simulink model "Mrinal_230929228_Simulink"  (R2025a)
settings: Solver=VariableStepAuto  StartTime=0.0  StopTime=5  RelTol=1e-3
libraries: spsSeriesRLCBranchLib x12, spsMeanLib x11, spsCurrentMeasurementLib x7, spsDCVoltageSourceLib x5, spsVoltageMeasurementLib x5, spsIdealSwitchLib x4, spspowerguiLib x4, spsDiodeLib x3, simulink x1, sps_lib x1
settings Model: Creator=MRINAL  LastModifiedBy=MRINAL

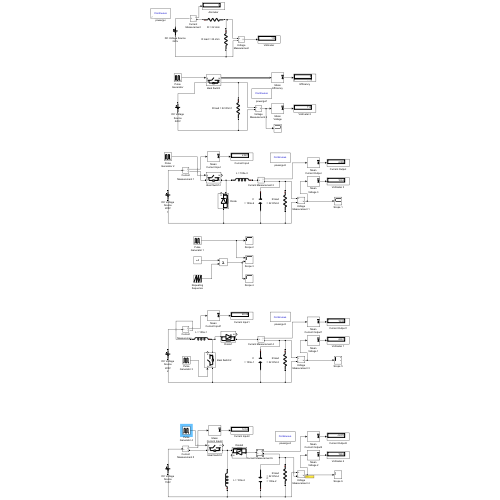
[thumbnail: Simulink's stored preview of the top-level diagram]
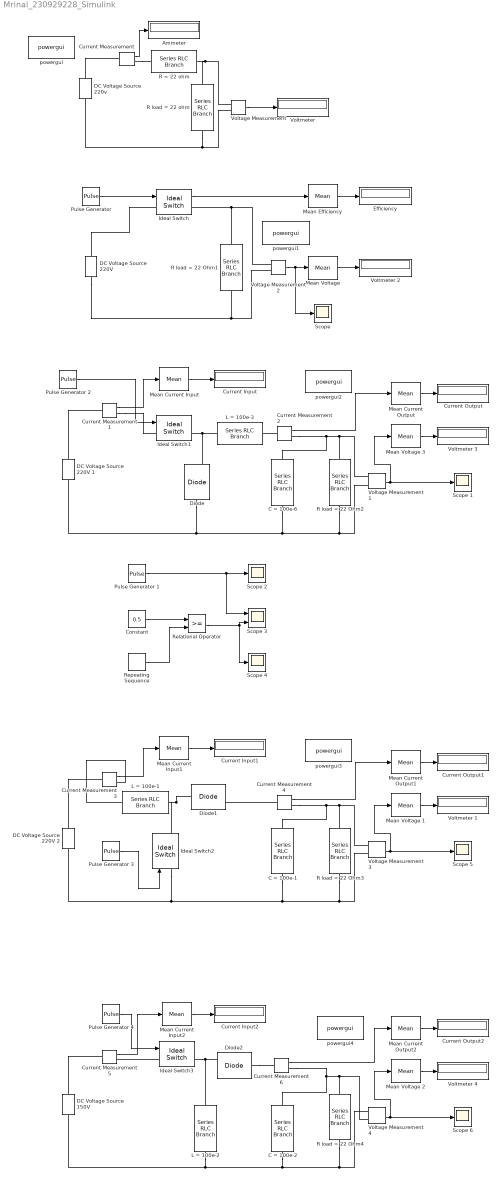
== system Mrinal_230929228_Simulink ==
  Ammeter : Display
  C = 100e-1 : spsSeriesRLCBranchLib/Series RLC Branch  LConnTagsString=__new0  RConnTagsString=__new0  BranchType=C  Resistance=22  Inductance=1e-3  SetiL0=off  InitialCurrent=0  Capacitance=100e-6  Setx0=off  InitialVoltage=0  Measurements=None
  C = 100e-2 : spsSeriesRLCBranchLib/Series RLC Branch  LConnTagsString=__new0  RConnTagsString=__new0  BranchType=C  Resistance=22  Inductance=1e-3  SetiL0=off  InitialCurrent=0  Capacitance=100e-6  Setx0=off  InitialVoltage=0  Measurements=None
  C = 100e-6 : spsSeriesRLCBranchLib/Series RLC Branch  LConnTagsString=__new0  RConnTagsString=__new0  BranchType=C  Resistance=22  Inductance=1e-3  SetiL0=off  InitialCurrent=0  Capacitance=100e-6  Setx0=off  InitialVoltage=0  Measurements=None
  Constant : Constant  Value=0.5
  Current Measurement : spsCurrentMeasurementLib/Current Measurement  PhasorSimulation=off  OutputType=Complex  PSBequivalent=0
  Current Measurement {1..6} (6 alike) : spsCurrentMeasurementLib/Current Measurement  PhasorSimulation=off  OutputType=Complex  PSBequivalent=0
  Current Input : Display
  Current Input1 : Display
  Current Input2 : Display
  Current Output : Display
  Current Output1 : Display
  Current Output2 : Display
  DC Voltage Source 150V : spsDCVoltageSourceLib/DC Voltage Source  Amplitude=150  Measurements=None
  DC Voltage Source 220V : spsDCVoltageSourceLib/DC Voltage Source  Amplitude=220  Measurements=None
  DC Voltage Source 220V 1 : spsDCVoltageSourceLib/DC Voltage Source  Amplitude=220  Measurements=None
  DC Voltage Source 220V 2 : spsDCVoltageSourceLib/DC Voltage Source  Amplitude=220  Measurements=None
  DC Voltage Source 220v : spsDCVoltageSourceLib/DC Voltage Source  Amplitude=220  Measurements=None
  Diode : spsDiodeLib/Diode  Ron=0.001  Lon=0  Vf=0.8  IC=0  UseSnubber=0  Rs=500  Cs=250e-9  Measurements=on
  Diode1 : spsDiodeLib/Diode  Ron=0.001  Lon=0  Vf=0.8  IC=0  UseSnubber=0  Rs=500  Cs=250e-9  Measurements=on
  Diode2 : spsDiodeLib/Diode  Ron=0.001  Lon=0  Vf=0.8  IC=0  UseSnubber=0  Rs=500  Cs=250e-9  Measurements=on
  Efficiency : Display
  Ideal Switch{,1..3} (4 alike) : spsIdealSwitchLib/Ideal Switch  Ron=0.001  Lon=0  IC=0  Rs=1e5  Cs=inf  Measurements=on
  L = 100e-1 : spsSeriesRLCBranchLib/Series RLC Branch  LConnTagsString=__new0  RConnTagsString=__new0  BranchType=L  Resistance=22  Inductance=100e-3  SetiL0=off  InitialCurrent=0  Capacitance=1e-6  Setx0=off  InitialVoltage=0  Measurements=None
  L = 100e-2 : spsSeriesRLCBranchLib/Series RLC Branch  LConnTagsString=__new0  RConnTagsString=__new0  BranchType=L  Resistance=22  Inductance=100e-3  SetiL0=off  InitialCurrent=0  Capacitance=1e-6  Setx0=off  InitialVoltage=0  Measurements=None
  L = 100e-3 : spsSeriesRLCBranchLib/Series RLC Branch  LConnTagsString=__new0  RConnTagsString=__new0  BranchType=L  Resistance=22  Inductance=100e-3  SetiL0=off  InitialCurrent=0  Capacitance=1e-6  Setx0=off  InitialVoltage=0  Measurements=None
  Mean Current Input : spsMeanLib/Mean  Freq=1  Vinit=0  Ts=0
  Mean Current Input1 : spsMeanLib/Mean  Freq=1  Vinit=0  Ts=0
  Mean Current Input2 : spsMeanLib/Mean  Freq=1  Vinit=0  Ts=0
  Mean Current Output : spsMeanLib/Mean  Freq=1  Vinit=0  Ts=0
  Mean Current Output1 : spsMeanLib/Mean  Freq=1  Vinit=0  Ts=0
  Mean Current Output2 : spsMeanLib/Mean  Freq=1  Vinit=0  Ts=0
  Mean Efficiency : spsMeanLib/Mean  Freq=1  Vinit=0  Ts=0
  Mean Voltage : spsMeanLib/Mean  Freq=1  Vinit=0  Ts=0
  Mean Voltage 1 : spsMeanLib/Mean  Freq=1  Vinit=0  Ts=0
  Mean Voltage 2 : spsMeanLib/Mean  Freq=1  Vinit=0  Ts=0
  Mean Voltage 3 : spsMeanLib/Mean  Freq=1  Vinit=0  Ts=0
  Pulse Generator : DiscretePulseGenerator  PulseType=Time based  Period=1  PulseWidth=50
  Pulse Generator 1 : DiscretePulseGenerator  PulseType=Time based  Period=1  PulseWidth=50
  Pulse Generator 2 : DiscretePulseGenerator  PulseType=Time based  Period=1/10000  PulseWidth=50
  Pulse Generator 3 : DiscretePulseGenerator  PulseType=Time based  Period=1/10000  PulseWidth=50
  Pulse Generator 4 : DiscretePulseGenerator  PulseType=Time based  Period=1/10000  PulseWidth=57.2
  R = 22 ohm : spsSeriesRLCBranchLib/Series RLC Branch  LConnTagsString=__new0  RConnTagsString=__new0  BranchType=R  Resistance=22  Inductance=1e-3  SetiL0=off  InitialCurrent=0  Capacitance=1e-6  Setx0=off  InitialVoltage=0  Measurements=None
  R load = 22 Ohm{1..4} (4 alike) : spsSeriesRLCBranchLib/Series RLC Branch  LConnTagsString=__new0  RConnTagsString=__new0  BranchType=R  Resistance=22  Inductance=1e-3  SetiL0=off  InitialCurrent=0  Capacitance=1e-6  Setx0=off  InitialVoltage=0  Measurements=None
  R load = 22 ohm : spsSeriesRLCBranchLib/Series RLC Branch  LConnTagsString=__new0  RConnTagsString=__new0  BranchType=R  Resistance=22  Inductance=1e-3  SetiL0=off  InitialCurrent=0  Capacitance=1e-6  Setx0=off  InitialVoltage=0  Measurements=None
  Relational Operator : RelationalOperator  OutDataTypeStr=boolean  RndMeth=Simplest  InputSameDT=off
  Repeating Sequence : simulink/Sources/Repeating Sequence  rep_seq_t=[0 1]  rep_seq_y=[0 1]
  Scope : Scope
      settings: Title=230929228_Mrinal_Kumar  ActiveDisplayYMinimum=-20.850014468769672  ActiveDisplayYMaximum=240.98523684109071  YLabel=Voltage (V)
  Scope {1..2,4..6} (5 alike) : Scope
      Scope 1 settings: Title=230929228_Mrinal_Kumar  ActiveDisplayYMinimum=-14.232493933115496  ActiveDisplayYMaximum=128.0924453980395  YLabel=Voltage (V)
      Scope 2 settings: Title=230929228_Mrinal_Kumar  ActiveDisplayYMinimum=-14.232493933115496  ActiveDisplayYMaximum=128.0924453980395  YLabel=Voltage (V)  DataLoggingVariableName=ScopeData2
      Scope 4 settings: Title=230929228_Mrinal_Kumar  ActiveDisplayYMinimum=-14.232493933115496  ActiveDisplayYMaximum=128.0924453980395  YLabel=Voltage (V)  DataLoggingVariableName=ScopeData4
      Scope 5 settings: Title=230929228_Mrinal_Kumar  ActiveDisplayYMinimum=-55.524699135554435  ActiveDisplayYMaximum=499.72229221999004  YLabel=Voltage (V)  DataLoggingVariableName=ScopeData5
      Scope 6 settings: Title=230929228_Mrinal_Kumar  ActiveDisplayYMinimum=-12.681597141404673  ActiveDisplayYMaximum=112.67772446783168  YLabel=Voltage (V)  DataLoggingVariableName=ScopeData6
  Scope 3 : Scope  NumInputPorts=2
      settings: Title=230929228_Mrinal_Kumar  ActiveDisplayYMinimum=-0.12499999999999997  ActiveDisplayYMaximum=1.125  YLabel=Voltage (V)  DataLoggingVariableName=ScopeData3
  Voltage Measurement : spsVoltageMeasurementLib/Voltage Measurement  PhasorSimulation=off  OutputType=Complex  PSBequivalent=0
  Voltage Measurement {1..4} (4 alike) : spsVoltageMeasurementLib/Voltage Measurement  PhasorSimulation=off  OutputType=Complex  PSBequivalent=0
  Voltmeter : Display
  Voltmeter {1..4} (4 alike) : Display
  powergui : sps_lib/powergui  Priority=1  SimulationMode=Continuous  SampleTime=50e-6  frequency=60  Iterations=50  frequencyindice=0  Pbase=100e6  ErrMax=1e-4  UnitsV=kV  UnitsW=MW  buscounter=0  FunctionMessages=off  echomessages=off  EnableUseOfTLC=off  CurrentSourceSwitches=off  DisableSnubberDevices=off  DisableRonSwitches=off  DisableVfSwitches=off  DisplayEquations=off  AutomaticDiscreteSolvers=off  SolverType=Tustin/Backward Euler (TBE)  Interpol=off  ExternalGateDelay=off  methode=off  Ts=100  x0status=zero  SPID=on  SwTol=0  HookPort=off  NonlinearTolerance=1e-4  nMaxIteration=100  ContinueOnMaxIteration=off  RestoreLinks=warning  ResistiveCurrentMeasurement=off  Frange=[0:2:500]  Ylog=off  Xlog=on  ShowGrid=off  save=off  variable=ZData  structure=0  ZoomFFT=off  StartTime=0.0  cycles=1  DisplayStyle=1  fundamental=60  FreqAxis=off  MaxFrequency=1000  frequencyindicesteady=1  RmsSteady=1  display=off
  powergui{1..4} (4 alike) : spspowerguiLib/powergui  Priority=1  SimulationMode=Continuous  SampleTime=50e-6  frequency=60  Iterations=50  frequencyindice=0  Pbase=100e6  ErrMax=1e-4  UnitsV=kV  UnitsW=MW  buscounter=0  FunctionMessages=off  echomessages=off  EnableUseOfTLC=off  CurrentSourceSwitches=off  DisableSnubberDevices=off  DisableRonSwitches=off  DisableVfSwitches=off  DisplayEquations=off  AutomaticDiscreteSolvers=off  SolverType=Tustin/Backward Euler (TBE)  Interpol=off  ExternalGateDelay=off  methode=off  Ts=100  x0status=zero  SPID=on  SwTol=0  HookPort=off  NonlinearTolerance=1e-4  nMaxIteration=100  ContinueOnMaxIteration=off  RestoreLinks=warning  ResistiveCurrentMeasurement=off  Frange=[0:2:500]  Ylog=off  Xlog=on  ShowGrid=off  save=off  variable=ZData  structure=0  ZoomFFT=off  StartTime=0.0  cycles=1  DisplayStyle=1  fundamental=60  FreqAxis=off  MaxFrequency=1000  frequencyindicesteady=1  RmsSteady=1  display=off
  wires:
  Current Measurement/1 -> Ammeter/1
  Voltage Measurement/1 -> Voltmeter/1
  Mean Voltage/1 -> Voltmeter 2/1
  Mean Efficiency/1 -> Efficiency/1
  Pulse Generator/1 -> Ideal Switch/1
  Ideal Switch/1 -> Mean Efficiency/1
  Voltage Measurement 2/1 -> Scope/1, Mean Voltage/1
  Current Measurement 1/1 -> Mean Current Input/1
  Mean Current Input/1 -> Current Input/1
  Pulse Generator 2/1 -> Ideal Switch1/1
  Current Measurement 2/1 -> Mean Current Output/1
  Mean Current Output/1 -> Current Output/1
  Mean Voltage 3/1 -> Voltmeter 3/1
  Voltage Measurement 1/1 -> Mean Voltage 3/1, Scope 1/1
  Repeating Sequence/1 -> Relational Operator/2
  Constant/1 -> Relational Operator/1
  Pulse Generator 1/1 -> Scope 2/1, Scope 3/1
  Relational Operator/1 -> Scope 4/1, Scope 3/2
  Mean Current Output1/1 -> Current Output1/1
  Mean Voltage 1/1 -> Voltmeter 1/1
  Voltage Measurement 3/1 -> Mean Voltage 1/1, Scope 5/1
  Mean Current Input1/1 -> Current Input1/1
  Current Measurement 4/1 -> Mean Current Output1/1
  Pulse Generator 3/1 -> Ideal Switch2/1
  Current Measurement 3/1 -> Mean Current Input1/1
  Current Measurement 6/1 -> Mean Current Output2/1
  Mean Voltage 2/1 -> Voltmeter 4/1
  Mean Current Output2/1 -> Current Output2/1
  Mean Current Input2/1 -> Current Input2/1
  Pulse Generator 4/1 -> Ideal Switch3/1
  Voltage Measurement 4/1 -> Mean Voltage 2/1, Scope 6/1
  Current Measurement 5/1 -> Mean Current Input2/1
  connections:
  DC Voltage Source 220v/RConn1 -- Current Measurement/LConn1
  Current Measurement/RConn1 -- R = 22 ohm/LConn1
  Voltage Measurement/LConn1 -- R load = 22 ohm/LConn1 -- R = 22 ohm/RConn1
  R load = 22 ohm/RConn1 -- DC Voltage Source 220v/LConn1 -- Voltage Measurement/LConn2
  R load = 22 Ohm1/LConn1 -- Voltage Measurement 2/LConn1 -- Ideal Switch/RConn1
  Ideal Switch/LConn1 -- DC Voltage Source 220V/RConn1
  DC Voltage Source 220V/LConn1 -- R load = 22 Ohm1/RConn1 -- Voltage Measurement 2/LConn2
  DC Voltage Source 220V 1/RConn1 -- Current Measurement 1/LConn1
  Current Measurement 1/RConn1 -- Ideal Switch1/LConn1
  L = 100e-3/RConn1 -- Diode/RConn1 -- Ideal Switch1/RConn1
  Current Measurement 2/LConn1 -- L = 100e-3/LConn1
  Current Measurement 2/RConn1 -- C = 100e-6/LConn1 -- R load = 22 Ohm2/LConn1 -- Voltage Measurement 1/LConn1
  C = 100e-6/RConn1 -- Diode/LConn1 -- DC Voltage Source 220V 1/LConn1 -- Voltage Measurement 1/LConn2 -- R load = 22 Ohm2/RConn1
  C = 100e-1/RConn1 -- Voltage Measurement 3/LConn2 -- R load = 22 Ohm3/RConn1 -- Ideal Switch2/LConn1 -- DC Voltage Source 220V 2/LConn1
  Voltage Measurement 3/LConn1 -- R load = 22 Ohm3/LConn1 -- Current Measurement 4/RConn1 -- C = 100e-1/LConn1
  DC Voltage Source 220V 2/RConn1 -- Current Measurement 3/LConn1
  L = 100e-1/RConn1 -- Current Measurement 3/RConn1
  Ideal Switch2/RConn1 -- Diode1/LConn1 -- L = 100e-1/LConn1
  Current Measurement 4/LConn1 -- Diode1/RConn1
  R load = 22 Ohm4/RConn1 -- Voltage Measurement 4/LConn1 -- DC Voltage Source 150V/LConn1 -- L = 100e-2/LConn1 -- C = 100e-2/LConn1
  Ideal Switch3/RConn1 -- L = 100e-2/RConn1 -- Diode2/RConn1
  Current Measurement 6/RConn1 -- C = 100e-2/RConn1 -- R load = 22 Ohm4/LConn1 -- Voltage Measurement 4/LConn2
  Ideal Switch3/LConn1 -- Current Measurement 5/RConn1
  DC Voltage Source 150V/RConn1 -- Current Measurement 5/LConn1
  Diode2/LConn1 -- Current Measurement 6/LConn1
